simulink model "controller"  (R2018a)
settings: Solver=FixedStepDiscrete  StartTime=0.0  StopTime=Inf  FixedStep=0.02  RelTol=1e-3  EnableMultiTasking=on
values from neighbouring files (symbols this model uses):
  DESTINATION_RANGE = 0.15    [controller_ws.mat]
  ENTRENCHED_MOTION = 3    [controller_ws.mat]
  FREE_MOTION = 1    [controller_ws.mat]
  MAX_ANGULAR_VELOCITY = 0.7    [controller_ws.mat]
  MAX_LINEAR_VELOCITY = 0.15    [controller_ws.mat]
  NO_VALUE = -60    [controller_ws.mat]
undefined symbols (not defined in the file or in its folder): Angular, Linear
libraries: simulink x11, robotlib x4
settings Model: Creator=The MathWorks, Inc.  LastModifiedBy=silviobacci
settings DataIOCC: LimitDataPoints=on  SaveFormat=Array
settings OptimizationCC: LifeSpan=Inf  MaxStackSize=64
settings DebuggingCC: SolverPrmCheckMsg=warning  AllowSymbolicDim=off  SFUnexpectedBacktrackingDiag=warning  SFNoUnconditionalDefaultTransitionDiag=warning  SFExecutionAtInitializationDiag=none
settings HardwareCC: ProdBitPerPointer=32  ProdBitPerSizeT=32  ProdBitPerPtrDiffT=32  ProdLargestAtomicFloat=None  ProdIntDivRoundTo=Undefined  ProdEndianess=Unspecified  ProdWordSize=32  ProdHWDeviceType=Generic->Unspecified (assume 32-bit Generic)  TargetHWDeviceType=Generic->Unspecified (assume 32-bit Generic)  UseEmbeddedCoderFeatures=off
settings ModelReferenceCC: PropagateSignalLabelsOutOfModel=off
settings RTWCC: SystemTargetFile=ert.tlc  HardwareBoard=Robot Operating System (ROS)  TemplateMakefile=ert_default_tmf  Toolchain=Catkin  TargetLang=C++
settings CodeAppCC: StateflowObjectComments=on
settings ERTTargetCC: MultiwordLength=2048  ERTCustomFileBanners=off  MultiInstanceERTCode=on  CodeInterfacePackaging=C++ class  SupportContinuousTime=on  SupportNonInlinedSFcns=on  RemoveResetFunc=off  SupportVariableSizeSignals=on  ModelStepFunctionPrototypeControlCompliant=off  RootIOFormat=Structure reference  ConvertIfToSwitch=off  SuppressUnreachableDefaultCases=off
settings ConfigComp: CovMetricSettings=dw  CovHtmlReporting=on  CovSaveCumulativeToWorkspaceVar=on  CovSaveSingleToWorkspaceVar=on  CovExternalEMLEnable=off  CovSFcnEnable=off

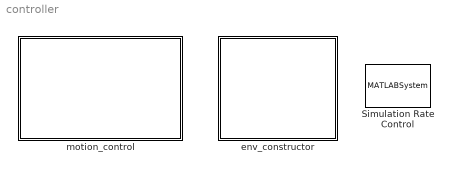
== system controller ==
  Simulation Rate Control : MATLABSystem  System=ExampleHelperSimulationRateControl  SampleTime=0.02
      mask Type: ExampleHelperSimulationRateControl
      mask Display: disp('Rate Control');
  env_constructor : Subsystem
  motion_control : Subsystem

== system controller/env_constructor ==
  Subscribe : robotlib/Subscribe  SourceLibraryInfo=This block requires Robotics System Toolbox  topicSource=Select from ROS network  topic=/env_constructor  messageType=turtlebot3_environment_scanner/tb_cloud_points  sampleTime=-1  messageQueueLength=1
      settings: SourceProductBaseCode=RO
  Subsystem : Subsystem
  wires:
  Subscribe/1 -> Subsystem/Enable
  Subscribe/2 -> Subsystem/1(tb_cloud_points)

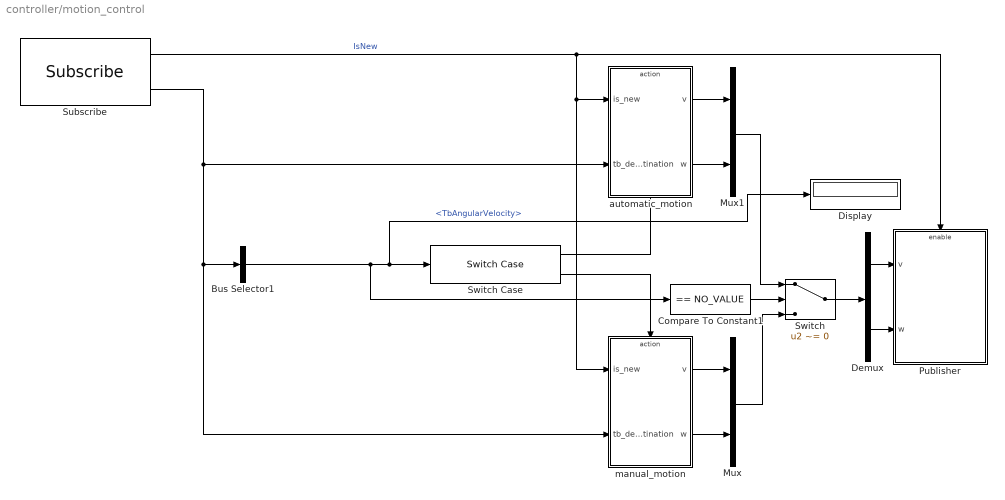
== system controller/motion_control ==
  Bus Selector1 : BusSelector  OutputSignals=TbAngularVelocity
  Compare To Constant1 : simulink/Logic and Bit Operations/Compare To Constant  relop===  const=NO_VALUE  OutDataTypeStr=boolean
  Demux : Demux  Outputs=2
  Display : Display
  Mux : Mux  Inputs=2
  Mux1 : Mux  Inputs=2
  Publisher : Subsystem
  Subscribe : robotlib/Subscribe  SourceLibraryInfo=This block requires Robotics System Toolbox  topicSource=Select from ROS network  topic=/tb_destination  messageType=turtlebot3_environment_scanner/tb_destination  sampleTime=-1  messageQueueLength=51
      settings: SourceProductBaseCode=RO
  Switch : Switch  Criteria=u2 ~= 0
  Switch Case : SwitchCase  CaseConditions={NO_VALUE}
  automatic_motion : Subsystem
  manual_motion : Subsystem
  wires:
  Subscribe/1 -> manual_motion/1(is_new), automatic_motion/1(is_new), Publisher/Enable  "IsNew"
  Subscribe/2 -> Bus Selector1/1, manual_motion/2(tb_destination), automatic_motion/2(tb_destination)
  Bus Selector1/1 -> Display/1, Switch Case/1, Compare To Constant1/1  "<TbAngularVelocity>"
  manual_motion/1(v) -> Mux/1
  manual_motion/2(w) -> Mux/2
  automatic_motion/1(v) -> Mux1/1
  automatic_motion/2(w) -> Mux1/2
  Demux/2 -> Publisher/2(w)
  Switch/1 -> Demux/1
  Compare To Constant1/1 -> Switch/2
  Switch Case/1 -> automatic_motion/Action
  Switch Case/2 -> manual_motion/Action
  Demux/1 -> Publisher/1(v)
  Mux1/1 -> Switch/1
  Mux/1 -> Switch/3

== system controller/env_constructor/Subsystem ==
  tb_cloud_points : Inport
  Enable : EnablePort
  Bus Selector : BusSelector  OutputSignals=TbX,TbY,CloudX,CloudY
  MATLAB Function : MATLAB Function  TreatAsAtomicUnit=on
  wires:
  Bus Selector/1 -> MATLAB Function/1(tb_x)  "<TbX>"
  Bus Selector/2 -> MATLAB Function/2(tb_y)  "<TbY>"
  tb_cloud_points/1 -> Bus Selector/1
  Bus Selector/3 -> MATLAB Function/3(cloud_x)  "<CloudX>"
  Bus Selector/4 -> MATLAB Function/4(cloud_y)  "<CloudY>"

== system controller/motion_control/Publisher ==
  v : Inport
  w : Inport  Port=2
  Enable : EnablePort
  Blank Message : robotlib/Blank Message  SourceLibraryInfo=This block requires Robotics System Toolbox  messageType=geometry_msgs/Twist  SampleTime=inf
      settings: SourceProductBaseCode=RO
  Bus Assignment1 : BusAssignment  DialogController=Simulink.DDGSource_BusAssignment  AssignedSignals=Linear.X,Angular.Z
  Publish2 : robotlib/Publish  SourceLibraryInfo=This block requires Robotics System Toolbox  topicSource=Select from ROS network  topic=/cmd_vel  messageType=geometry_msgs/Twist  messageQueueLength=105
      settings: SourceProductBaseCode=RO
  wires:
  Bus Assignment1/1 -> Publish2/1
  Blank Message/1 -> Bus Assignment1/1
  v/1 -> Bus Assignment1/2
  w/1 -> Bus Assignment1/3

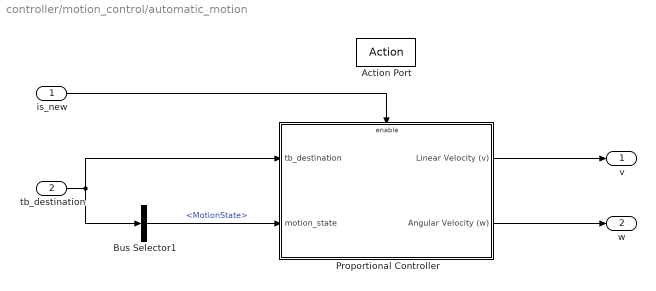
== system controller/motion_control/automatic_motion ==
  is_new : Inport
  tb_destination : Inport  Port=2
  Action Port : ActionPort  ActionType=case
  Bus Selector1 : BusSelector  OutputSignals=MotionState
  Proportional Controller : Subsystem
  v : Outport
  w : Outport  Port=2
  wires:
  Proportional Controller/2(Angular Velocity (w)) -> w/1
  Proportional Controller/1(Linear Velocity (v)) -> v/1
  is_new/1 -> Proportional Controller/Enable
  tb_destination/1 -> Proportional Controller/1(tb_destination), Bus Selector1/1
  Bus Selector1/1 -> Proportional Controller/2(motion_state)  "<MotionState>"

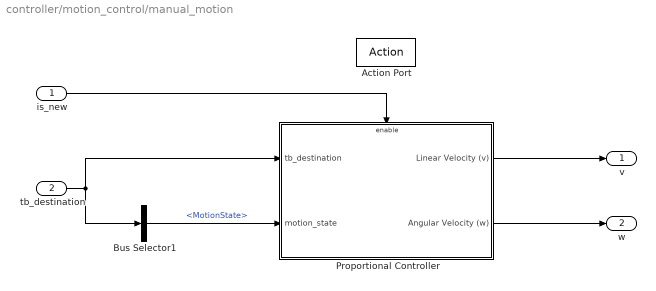
== system controller/motion_control/manual_motion ==
  is_new : Inport
  tb_destination : Inport  Port=2
  Action Port : ActionPort  ActionType=default
  Bus Selector1 : BusSelector  OutputSignals=MotionState
  Proportional Controller : Subsystem
  v : Outport
  w : Outport  Port=2
  wires:
  Proportional Controller/2(Angular Velocity (w)) -> w/1
  Proportional Controller/1(Linear Velocity (v)) -> v/1
  is_new/1 -> Proportional Controller/Enable
  tb_destination/1 -> Proportional Controller/1(tb_destination), Bus Selector1/1
  Bus Selector1/1 -> Proportional Controller/2(motion_state)  "<MotionState>"

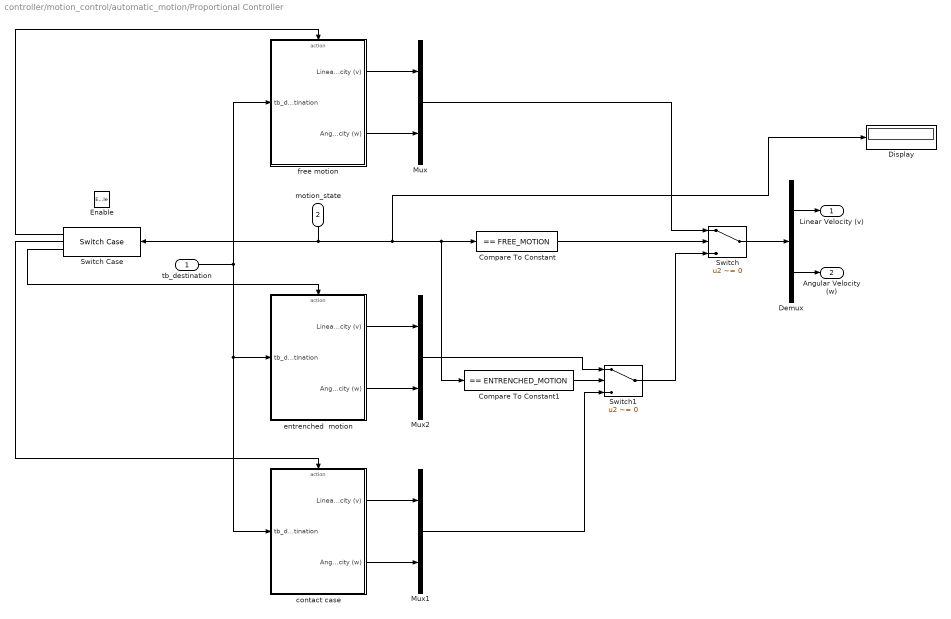
== system controller/motion_control/automatic_motion/Proportional Controller ==
  tb_destination : Inport
  motion_state : Inport  Port=2
  Enable : EnablePort
  Compare To Constant : simulink/Logic and Bit Operations/Compare To Constant  relop===  const=FREE_MOTION  OutDataTypeStr=boolean
  Compare To Constant1 : simulink/Logic and Bit Operations/Compare To Constant  relop===  const=ENTRENCHED_MOTION  OutDataTypeStr=boolean
  Demux : Demux  Outputs=2
  Display : Display
  Mux : Mux  Inputs=2
  Mux1 : Mux  Inputs=2
  Mux2 : Mux  Inputs=2
  Switch : Switch  Criteria=u2 ~= 0
  Switch Case : SwitchCase  CaseConditions={FREE_MOTION, CONTACT_MOTION, ENTRENCHED_MOTION}  ShowDefaultCase=off
  Switch1 : Switch  Criteria=u2 ~= 0
  contact case : Subsystem
  entrenched  motion : Subsystem
  free motion : Subsystem
  Linear Velocity (v) : Outport
  Angular Velocity (w) : Outport  Port=2
  wires:
  motion_state/1 -> Switch Case/1, Display/1, Compare To Constant1/1, Compare To Constant/1
  Switch Case/1 -> free motion/Action
  Switch Case/3 -> entrenched  motion/Action
  free motion/1(Linear Velocity (v)) -> Mux/1
  free motion/2(Angular Velocity (w)) -> Mux/2
  Demux/1 -> Linear Velocity (v)/1
  Demux/2 -> Angular Velocity (w)/1
  Compare To Constant/1 -> Switch/2
  Mux/1 -> Switch/1
  Switch/1 -> Demux/1
  Compare To Constant1/1 -> Switch1/2
  Switch1/1 -> Switch/3
  Switch Case/2 -> contact case/Action
  contact case/1(Linear Velocity (v)) -> Mux1/1
  contact case/2(Angular Velocity (w)) -> Mux1/2
  entrenched  motion/1(Linear Velocity (v)) -> Mux2/1
  entrenched  motion/2(Angular Velocity (w)) -> Mux2/2
  Mux2/1 -> Switch1/1
  Mux1/1 -> Switch1/3
  tb_destination/1 -> free motion/1(tb_destination), entrenched  motion/1(tb_destination), contact case/1(tb_destination)

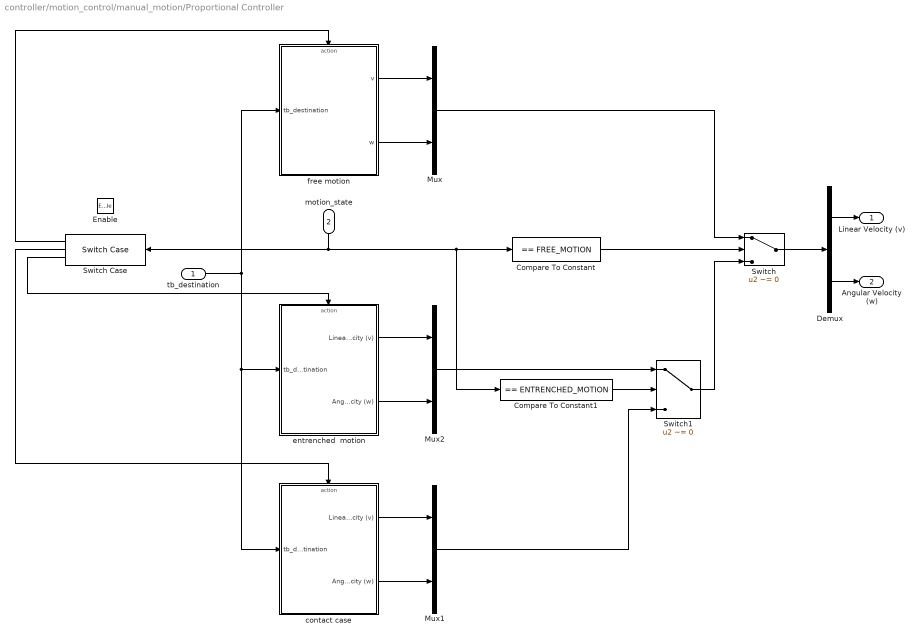
== system controller/motion_control/manual_motion/Proportional Controller ==
  tb_destination : Inport
  motion_state : Inport  Port=2
  Enable : EnablePort
  Compare To Constant : simulink/Logic and Bit Operations/Compare To Constant  relop===  const=FREE_MOTION  OutDataTypeStr=boolean
  Compare To Constant1 : simulink/Logic and Bit Operations/Compare To Constant  relop===  const=ENTRENCHED_MOTION  OutDataTypeStr=boolean
  Demux : Demux  Outputs=2
  Mux : Mux  Inputs=2
  Mux1 : Mux  Inputs=2
  Mux2 : Mux  Inputs=2
  Switch : Switch  Criteria=u2 ~= 0
  Switch Case : SwitchCase  CaseConditions={FREE_MOTION, CONTACT_MOTION, ENTRENCHED_MOTION}  ShowDefaultCase=off
  Switch1 : Switch  Criteria=u2 ~= 0
  contact case : Subsystem
  entrenched  motion : Subsystem
  free motion : Subsystem
  Linear Velocity (v) : Outport
  Angular Velocity (w) : Outport  Port=2
  wires:
  motion_state/1 -> Switch Case/1, Compare To Constant1/1, Compare To Constant/1
  Switch Case/1 -> free motion/Action
  Switch Case/3 -> entrenched  motion/Action
  free motion/1(v) -> Mux/1
  free motion/2(w) -> Mux/2
  Demux/1 -> Linear Velocity (v)/1
  Demux/2 -> Angular Velocity (w)/1
  Compare To Constant/1 -> Switch/2
  Mux/1 -> Switch/1
  Switch/1 -> Demux/1
  Compare To Constant1/1 -> Switch1/2
  Switch1/1 -> Switch/3
  Switch Case/2 -> contact case/Action
  contact case/1(Linear Velocity (v)) -> Mux1/1
  contact case/2(Angular Velocity (w)) -> Mux1/2
  entrenched  motion/1(Linear Velocity (v)) -> Mux2/1
  entrenched  motion/2(Angular Velocity (w)) -> Mux2/2
  tb_destination/1 -> contact case/1(tb_destination), entrenched  motion/1(tb_destination), free motion/1(tb_destination)
  Mux1/1 -> Switch1/3
  Mux2/1 -> Switch1/1

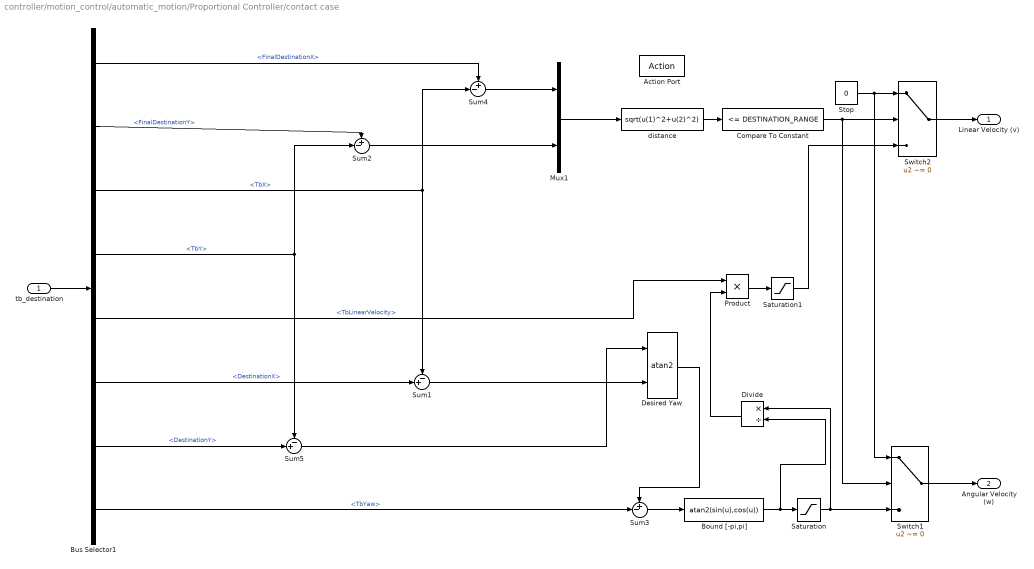
== system controller/motion_control/automatic_motion/Proportional Controller/contact case ==
  tb_destination : Inport
  Action Port : ActionPort  ActionType=case
  Bound [-pi,pi] : Fcn  Expr=atan2(sin(u),cos(u))
  Bus Selector1 : BusSelector  OutputSignals=FinalDestinationX,FinalDestinationY,TbX,TbY,TbLinearVelocity,DestinationX,DestinationY,TbYaw
  Compare To Constant : simulink/Logic and Bit Operations/Compare To Constant  relop=<=  const=DESTINATION_RANGE  OutDataTypeStr=boolean
  Desired Yaw : Trigonometry  Operator=atan2
  Divide : Product  Inputs=*/
  Mux1 : Mux  Inputs=2
  Product : Product
  Saturation : Saturate  UpperLimit=MAX_ANGULAR_VELOCITY  LowerLimit=-MAX_ANGULAR_VELOCITY
  Saturation1 : Saturate  UpperLimit=MAX_LINEAR_VELOCITY  LowerLimit=-MAX_LINEAR_VELOCITY
  Stop : Constant  Value=0
  Sum1 : Sum  Inputs=-+|
  Sum2 : Sum  Inputs=+-|
  Sum3 : Sum  Inputs=+-|
  Sum4 : Sum  Inputs=+-|
  Sum5 : Sum  Inputs=-+|
  Switch1 : Switch  Criteria=u2 ~= 0
  Switch2 : Switch  Criteria=u2 ~= 0
  distance : Fcn  Expr=sqrt(u(1)^2+u(2)^2)
  Linear Velocity (v) : Outport
  Angular Velocity (w) : Outport  Port=2
  wires:
  distance/1 -> Compare To Constant/1
  Switch1/1 -> Angular Velocity (w)/1
  Bus Selector1/5 -> Product/1  "<TbLinearVelocity>"
  tb_destination/1 -> Bus Selector1/1
  Sum2/1 -> Mux1/2
  Bus Selector1/6 -> Sum1/2  "<DestinationX>"
  Bus Selector1/7 -> Sum5/2  "<DestinationY>"
  Switch2/1 -> Linear Velocity (v)/1
  Stop/1 -> Switch1/1, Switch2/1
  Desired Yaw/1 -> Sum3/1
  Mux1/1 -> distance/1
  Sum4/1 -> Mux1/1
  Compare To Constant/1 -> Switch2/2, Switch1/2
  Bus Selector1/4 -> Sum2/2, Sum5/1  "<TbY>"
  Bus Selector1/3 -> Sum4/2, Sum1/1  "<TbX>"
  Bus Selector1/1 -> Sum4/1  "<FinalDestinationX>"
  Bus Selector1/2 -> Sum2/1  "<FinalDestinationY>"
  Sum5/1 -> Desired Yaw/1
  Sum1/1 -> Desired Yaw/2
  Saturation1/1 -> Switch2/3
  Product/1 -> Saturation1/1
  Bound [-pi,pi]/1 -> Saturation/1, Divide/2
  Saturation/1 -> Divide/1, Switch1/3
  Divide/1 -> Product/2
  Sum3/1 -> Bound [-pi,pi]/1
  Bus Selector1/8 -> Sum3/2  "<TbYaw>"

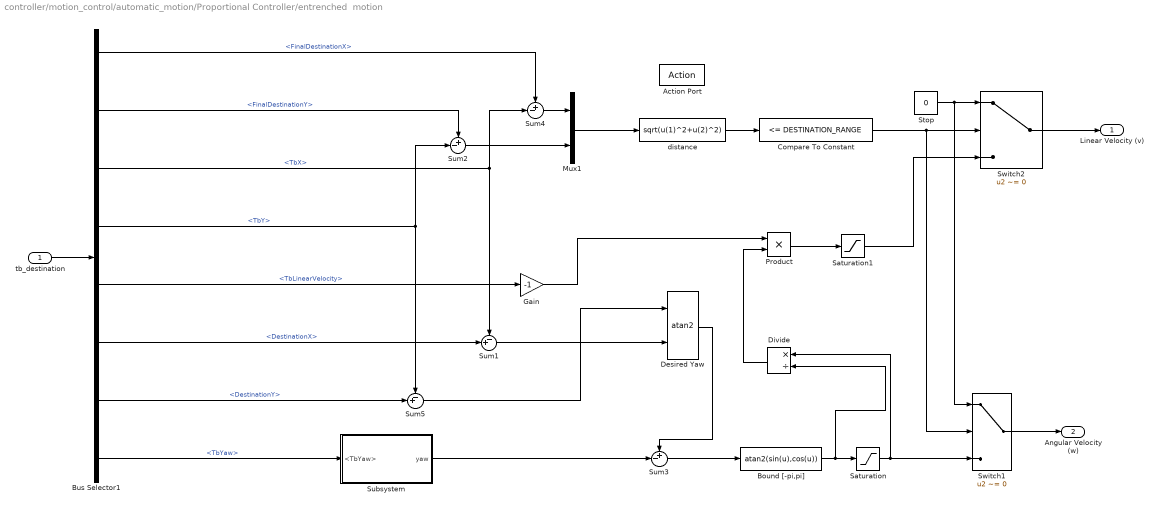
== system controller/motion_control/automatic_motion/Proportional Controller/entrenched  motion ==
  tb_destination : Inport
  Action Port : ActionPort  ActionType=case
  Bound [-pi,pi] : Fcn  Expr=atan2(sin(u),cos(u))
  Bus Selector1 : BusSelector  OutputSignals=FinalDestinationX,FinalDestinationY,TbX,TbY,TbLinearVelocity,DestinationX,DestinationY,TbYaw
  Compare To Constant : simulink/Logic and Bit Operations/Compare To Constant  relop=<=  const=DESTINATION_RANGE  OutDataTypeStr=boolean
  Desired Yaw : Trigonometry  Operator=atan2
  Divide : Product  Inputs=*/
  Gain : Gain  Gain=-1
  Mux1 : Mux  Inputs=2
  Product : Product
  Saturation : Saturate  UpperLimit=MAX_ANGULAR_VELOCITY  LowerLimit=-MAX_ANGULAR_VELOCITY
  Saturation1 : Saturate  UpperLimit=MAX_LINEAR_VELOCITY  LowerLimit=-MAX_LINEAR_VELOCITY
  Stop : Constant  Value=0
  Subsystem : Subsystem
  Sum1 : Sum  Inputs=-+|
  Sum2 : Sum  Inputs=+-|
  Sum3 : Sum  Inputs=+-|
  Sum4 : Sum  Inputs=+-|
  Sum5 : Sum  Inputs=-+|
  Switch1 : Switch  Criteria=u2 ~= 0
  Switch2 : Switch  Criteria=u2 ~= 0
  distance : Fcn  Expr=sqrt(u(1)^2+u(2)^2)
  Linear Velocity (v) : Outport
  Angular Velocity (w) : Outport  Port=2
  wires:
  Bus Selector1/2 -> Sum2/1  "<FinalDestinationY>"
  Bus Selector1/1 -> Sum4/1  "<FinalDestinationX>"
  Sum2/1 -> Mux1/2
  Switch2/1 -> Linear Velocity (v)/1
  Stop/1 -> Switch1/1, Switch2/1
  Desired Yaw/1 -> Sum3/1
  Sum5/1 -> Desired Yaw/1
  Sum4/1 -> Mux1/1
  Bus Selector1/7 -> Sum5/2  "<DestinationY>"
  tb_destination/1 -> Bus Selector1/1
  Compare To Constant/1 -> Switch2/2, Switch1/2
  distance/1 -> Compare To Constant/1
  Switch1/1 -> Angular Velocity (w)/1
  Sum3/1 -> Bound [-pi,pi]/1
  Sum1/1 -> Desired Yaw/2
  Bus Selector1/6 -> Sum1/2  "<DestinationX>"
  Mux1/1 -> distance/1
  Bus Selector1/4 -> Sum2/2, Sum5/1  "<TbY>"
  Bus Selector1/3 -> Sum4/2, Sum1/1  "<TbX>"
  Bus Selector1/8 -> Subsystem/1(<TbYaw>)  "<TbYaw>"
  Product/1 -> Saturation1/1
  Bound [-pi,pi]/1 -> Saturation/1, Divide/2
  Saturation/1 -> Divide/1, Switch1/3
  Divide/1 -> Product/2
  Saturation1/1 -> Switch2/3
  Bus Selector1/5 -> Gain/1  "<TbLinearVelocity>"
  Subsystem/1(yaw) -> Sum3/2
  Gain/1 -> Product/1

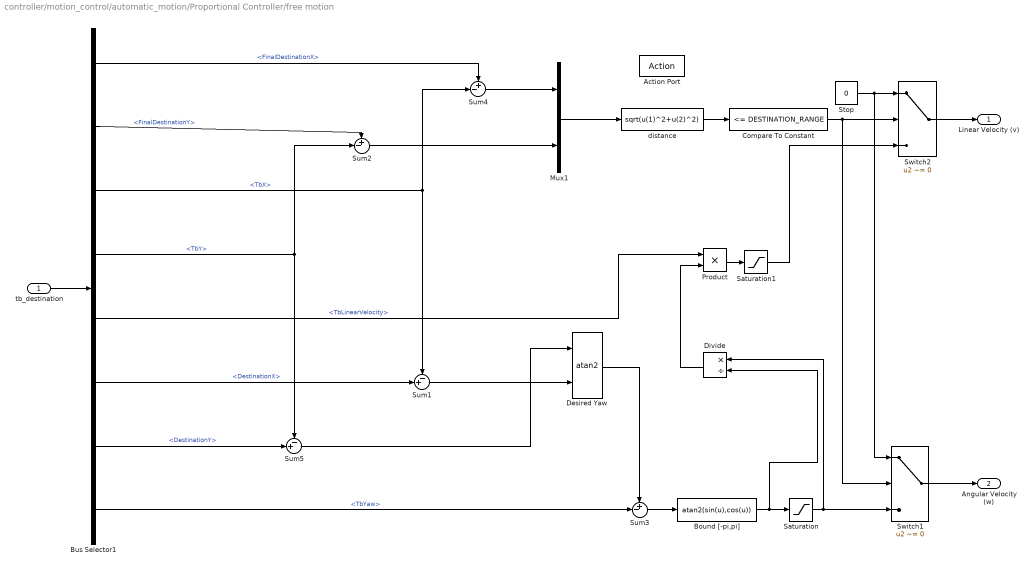
== system controller/motion_control/automatic_motion/Proportional Controller/free motion ==
  tb_destination : Inport
  Action Port : ActionPort  ActionType=case
  Bound [-pi,pi] : Fcn  Expr=atan2(sin(u),cos(u))
  Bus Selector1 : BusSelector  OutputSignals=FinalDestinationX,FinalDestinationY,TbX,TbY,TbLinearVelocity,DestinationX,DestinationY,TbYaw
  Compare To Constant : simulink/Logic and Bit Operations/Compare To Constant  relop=<=  const=DESTINATION_RANGE  OutDataTypeStr=boolean
  Desired Yaw : Trigonometry  Operator=atan2
  Divide : Product  Inputs=*/
  Mux1 : Mux  Inputs=2
  Product : Product
  Saturation : Saturate  UpperLimit=MAX_ANGULAR_VELOCITY  LowerLimit=-MAX_ANGULAR_VELOCITY
  Saturation1 : Saturate  UpperLimit=MAX_LINEAR_VELOCITY  LowerLimit=-MAX_LINEAR_VELOCITY
  Stop : Constant  Value=0
  Sum1 : Sum  Inputs=-+|
  Sum2 : Sum  Inputs=+-|
  Sum3 : Sum  Inputs=+-|
  Sum4 : Sum  Inputs=+-|
  Sum5 : Sum  Inputs=-+|
  Switch1 : Switch  Criteria=u2 ~= 0
  Switch2 : Switch  Criteria=u2 ~= 0
  distance : Fcn  Expr=sqrt(u(1)^2+u(2)^2)
  Linear Velocity (v) : Outport
  Angular Velocity (w) : Outport  Port=2
  wires:
  Switch1/1 -> Angular Velocity (w)/1
  Sum3/1 -> Bound [-pi,pi]/1
  Bus Selector1/2 -> Sum2/1  "<FinalDestinationY>"
  Sum5/1 -> Desired Yaw/1
  Stop/1 -> Switch1/1, Switch2/1
  Bus Selector1/7 -> Sum5/2  "<DestinationY>"
  Sum1/1 -> Desired Yaw/2
  Bus Selector1/4 -> Sum2/2, Sum5/1  "<TbY>"
  Compare To Constant/1 -> Switch2/2, Switch1/2
  Mux1/1 -> distance/1
  Bus Selector1/1 -> Sum4/1  "<FinalDestinationX>"
  Desired Yaw/1 -> Sum3/1
  Sum4/1 -> Mux1/1
  Bus Selector1/3 -> Sum4/2, Sum1/1  "<TbX>"
  Switch2/1 -> Linear Velocity (v)/1
  tb_destination/1 -> Bus Selector1/1
  Bus Selector1/6 -> Sum1/2  "<DestinationX>"
  Sum2/1 -> Mux1/2
  distance/1 -> Compare To Constant/1
  Bus Selector1/8 -> Sum3/2  "<TbYaw>"
  Saturation/1 -> Switch1/3, Divide/1
  Bound [-pi,pi]/1 -> Saturation/1, Divide/2
  Divide/1 -> Product/2
  Bus Selector1/5 -> Product/1  "<TbLinearVelocity>"
  Product/1 -> Saturation1/1
  Saturation1/1 -> Switch2/3

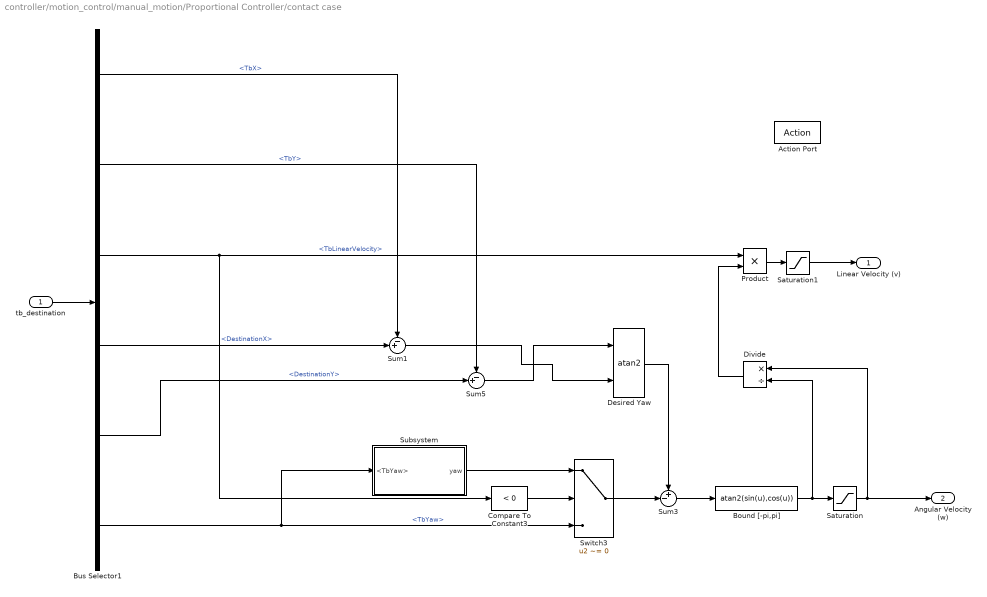
== system controller/motion_control/manual_motion/Proportional Controller/contact case ==
  tb_destination : Inport
  Action Port : ActionPort  ActionType=case
  Bound [-pi,pi] : Fcn  Expr=atan2(sin(u),cos(u))
  Bus Selector1 : BusSelector  OutputSignals=TbX,TbY,TbLinearVelocity,DestinationX,DestinationY,TbYaw
  Compare To Constant3 : simulink/Logic and Bit Operations/Compare To Constant  relop=<  const=0  OutDataTypeStr=boolean
  Desired Yaw : Trigonometry  Operator=atan2
  Divide : Product  Inputs=*/
  Product : Product
  Saturation : Saturate  UpperLimit=MAX_ANGULAR_VELOCITY  LowerLimit=-MAX_ANGULAR_VELOCITY
  Saturation1 : Saturate  UpperLimit=MAX_LINEAR_VELOCITY  LowerLimit=-MAX_LINEAR_VELOCITY
  Subsystem : Subsystem
  Sum1 : Sum  Inputs=-+|
  Sum3 : Sum  Inputs=+-|
  Sum5 : Sum  Inputs=-+|
  Switch3 : Switch  Criteria=u2 ~= 0
  Linear Velocity (v) : Outport
  Angular Velocity (w) : Outport  Port=2
  wires:
  Bus Selector1/6 -> Subsystem/1(<TbYaw>), Switch3/3  "<TbYaw>"
  Bus Selector1/5 -> Sum5/2  "<DestinationY>"
  Bus Selector1/4 -> Sum1/2  "<DestinationX>"
  Bus Selector1/1 -> Sum1/1  "<TbX>"
  tb_destination/1 -> Bus Selector1/1
  Desired Yaw/1 -> Sum3/1
  Switch3/1 -> Sum3/2
  Sum1/1 -> Desired Yaw/2
  Bus Selector1/3 -> Product/1, Compare To Constant3/1  "<TbLinearVelocity>"
  Bus Selector1/2 -> Sum5/1  "<TbY>"
  Compare To Constant3/1 -> Switch3/2
  Saturation/1 -> Angular Velocity (w)/1, Divide/1
  Sum5/1 -> Desired Yaw/1
  Subsystem/1(yaw) -> Switch3/1
  Product/1 -> Saturation1/1
  Sum3/1 -> Bound [-pi,pi]/1
  Bound [-pi,pi]/1 -> Saturation/1, Divide/2
  Divide/1 -> Product/2
  Saturation1/1 -> Linear Velocity (v)/1

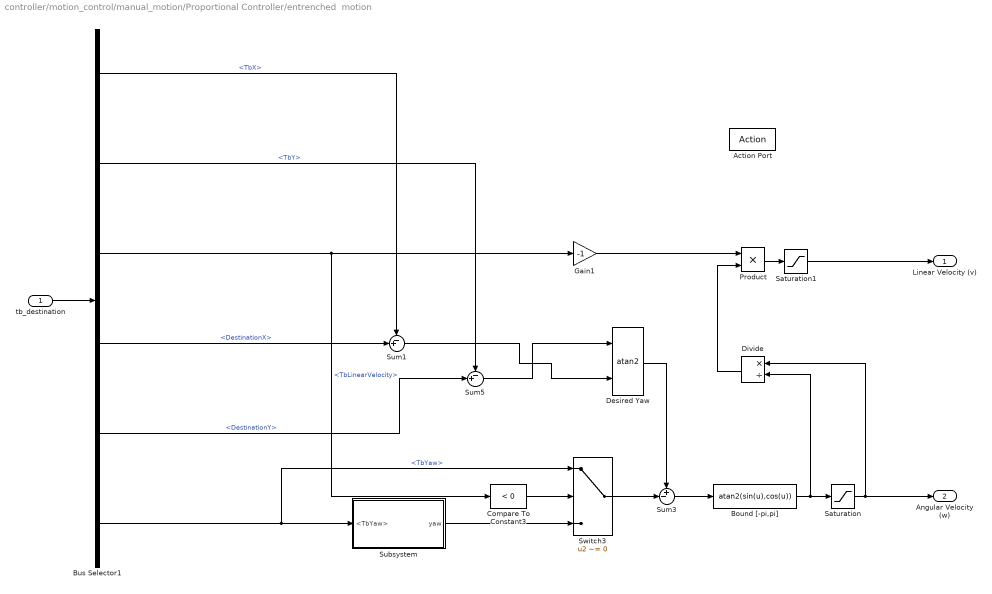
== system controller/motion_control/manual_motion/Proportional Controller/entrenched  motion ==
  tb_destination : Inport
  Action Port : ActionPort  ActionType=case
  Bound [-pi,pi] : Fcn  Expr=atan2(sin(u),cos(u))
  Bus Selector1 : BusSelector  OutputSignals=TbX,TbY,TbLinearVelocity,DestinationX,DestinationY,TbYaw
  Compare To Constant3 : simulink/Logic and Bit Operations/Compare To Constant  relop=<  const=0  OutDataTypeStr=boolean
  Desired Yaw : Trigonometry  Operator=atan2
  Divide : Product  Inputs=*/
  Gain1 : Gain  Gain=-1
  Product : Product
  Saturation : Saturate  UpperLimit=MAX_ANGULAR_VELOCITY  LowerLimit=-MAX_ANGULAR_VELOCITY
  Saturation1 : Saturate  UpperLimit=MAX_LINEAR_VELOCITY  LowerLimit=-MAX_LINEAR_VELOCITY
  Subsystem : Subsystem
  Sum1 : Sum  Inputs=-+|
  Sum3 : Sum  Inputs=+-|
  Sum5 : Sum  Inputs=-+|
  Switch3 : Switch  Criteria=u2 ~= 0
  Linear Velocity (v) : Outport
  Angular Velocity (w) : Outport  Port=2
  wires:
  Bus Selector1/6 -> Subsystem/1(<TbYaw>), Switch3/1  "<TbYaw>"
  Bus Selector1/2 -> Sum5/1  "<TbY>"
  Compare To Constant3/1 -> Switch3/2
  Desired Yaw/1 -> Sum3/1
  Bus Selector1/1 -> Sum1/1  "<TbX>"
  Bus Selector1/3 -> Compare To Constant3/1, Gain1/1  "<TbLinearVelocity>"
  Saturation/1 -> Angular Velocity (w)/1, Divide/1
  tb_destination/1 -> Bus Selector1/1
  Switch3/1 -> Sum3/2
  Subsystem/1(yaw) -> Switch3/3
  Bus Selector1/5 -> Sum5/2  "<DestinationY>"
  Bus Selector1/4 -> Sum1/2  "<DestinationX>"
  Sum5/1 -> Desired Yaw/1
  Sum1/1 -> Desired Yaw/2
  Product/1 -> Saturation1/1
  Sum3/1 -> Bound [-pi,pi]/1
  Bound [-pi,pi]/1 -> Saturation/1, Divide/2
  Divide/1 -> Product/2
  Saturation1/1 -> Linear Velocity (v)/1
  Gain1/1 -> Product/1

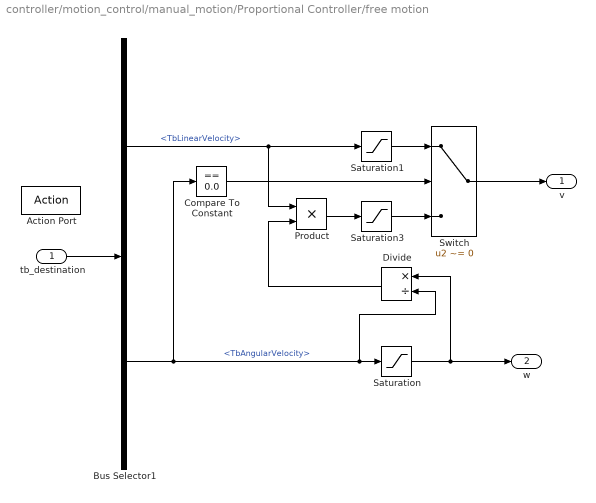
== system controller/motion_control/manual_motion/Proportional Controller/free motion ==
  tb_destination : Inport
  Action Port : ActionPort  ActionType=case
  Bus Selector1 : BusSelector  OutputSignals=TbLinearVelocity,TbAngularVelocity
  Compare To Constant : simulink/Logic and Bit Operations/Compare To Constant  relop===  const=0.0  OutDataTypeStr=boolean
  Divide : Product  Inputs=*/
  Product : Product
  Saturation : Saturate  UpperLimit=MAX_ANGULAR_VELOCITY  LowerLimit=-MAX_ANGULAR_VELOCITY
  Saturation1 : Saturate  UpperLimit=MAX_LINEAR_VELOCITY  LowerLimit=-MAX_LINEAR_VELOCITY
  Saturation3 : Saturate  UpperLimit=MAX_LINEAR_VELOCITY  LowerLimit=-MAX_LINEAR_VELOCITY
  Switch : Switch  Criteria=u2 ~= 0
  v : Outport
  w : Outport  Port=2
  wires:
  tb_destination/1 -> Bus Selector1/1
  Bus Selector1/2 -> Saturation/1, Divide/2, Compare To Constant/1  "<TbAngularVelocity>"
  Product/1 -> Saturation3/1
  Saturation/1 -> w/1, Divide/1
  Divide/1 -> Product/2
  Bus Selector1/1 -> Product/1, Saturation1/1  "<TbLinearVelocity>"
  Compare To Constant/1 -> Switch/2
  Switch/1 -> v/1
  Saturation3/1 -> Switch/3
  Saturation1/1 -> Switch/1

== system controller/motion_control/automatic_motion/Proportional Controller/entrenched  motion/Subsystem ==
  <TbYaw> : Inport
  Constant : Constant  Value=2 * pi
  Math Function : Math  Operator=mod  SaturateOnIntegerOverflow=on
  inverse orientation : Fcn  Expr=u + pi
  yaw : Outport
  wires:
  <TbYaw>/1 -> inverse orientation/1
  Math Function/1 -> yaw/1
  Constant/1 -> Math Function/2
  inverse orientation/1 -> Math Function/1

== system controller/motion_control/manual_motion/Proportional Controller/contact case/Subsystem ==
  <TbYaw> : Inport
  Constant : Constant  Value=2 * pi
  Math Function : Math  Operator=mod  SaturateOnIntegerOverflow=on
  inverse orientation : Fcn  Expr=u + pi
  yaw : Outport
  wires:
  <TbYaw>/1 -> inverse orientation/1
  Math Function/1 -> yaw/1
  Constant/1 -> Math Function/2
  inverse orientation/1 -> Math Function/1

== system controller/motion_control/manual_motion/Proportional Controller/entrenched  motion/Subsystem ==
  <TbYaw> : Inport
  Constant : Constant  Value=2 * pi
  Math Function : Math  Operator=mod  SaturateOnIntegerOverflow=on
  inverse orientation : Fcn  Expr=u + pi
  yaw : Outport
  wires:
  <TbYaw>/1 -> inverse orientation/1
  Math Function/1 -> yaw/1
  Constant/1 -> Math Function/2
  inverse orientation/1 -> Math Function/1

== matlab function controller/env_constructor/Subsystem/MATLAB Function ==
  data: tb_x input; tb_y input; cloud_x input; cloud_y input
function plot_environment(tb_x, tb_y, cloud_x, cloud_y)

coder.extrinsic('scatter')
scatter(-tb_y, tb_x, 20, 'red', 'filled');
scatter(-cloud_y, cloud_x, 10, 'black', 'filled');
xlim([-3, 3])
ylim([-3, 3])
hold on
